simulink model "twoturbine"  (R2015b)
settings: Solver=VariableStepAuto  StartTime=0.0  StopTime=25  RelTol=1e-3
undefined symbols (not defined in the file): Ts
libraries: powerlib_meascontrol x4, powerlib x3, GE_275_103 x2
settings Model: SimulationMode=accelerator  Creator=Eren  LastModifiedBy=Eren

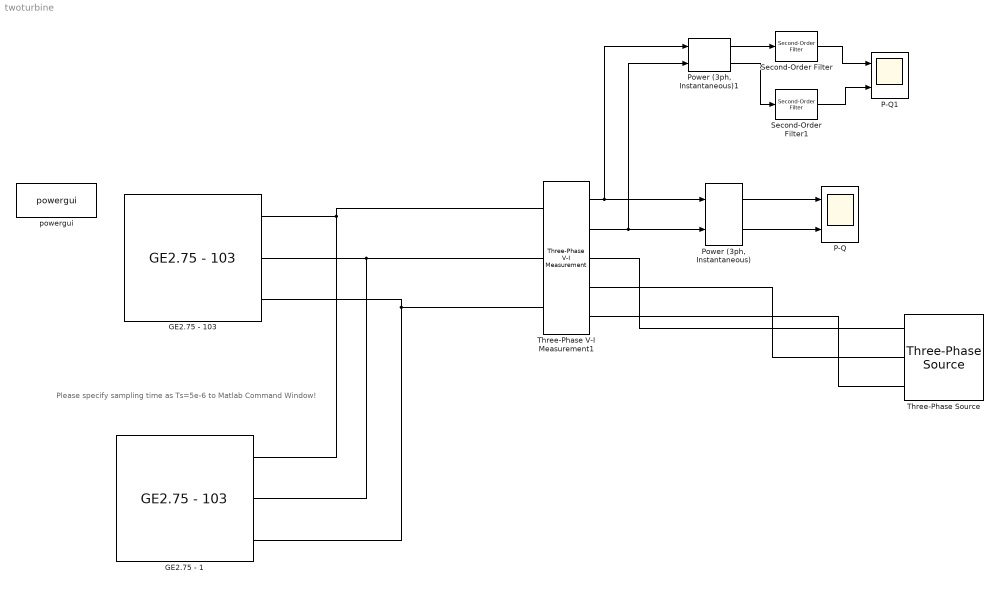
== system twoturbine ==
  note: Please specify sampling time as Ts=5e-6 to Matlab Command Window!
  GE2.75 - 1 : GE_275_103/GE2.75 - 103  Prated=2.75e6  R=51.5  windspeed=9  Jtotal=1058.2  p=1.225  startuptime=5  winit=-160  gear=117.4  wmax=2*pi*(1735/60)  fluxlinkage=4  pgen=2  Ld=10e-4  Lq=10.5e-4  Rs=1e-10  drivefreq=10e3  fnom=50  Srated=3.04e6  Vdcset=2500  Cdc=27e-3  Lfilter=2e-4
  GE2.75 - 103 : GE_275_103/GE2.75 - 103  Prated=2.75e6  R=51.5  windspeed=9  Jtotal=1058.2  p=1.225  startuptime=5  winit=-160  gear=117.4  wmax=2*pi*(1735/60)  fluxlinkage=4  pgen=2  Ld=10e-4  Lq=10.5e-4  Rs=1e-10  drivefreq=10e3  fnom=50  Srated=3.04e6  Vdcset=2500  Cdc=27e-3  Lfilter=2e-4
  P-Q : Scope  NumInputPorts=2
  P-Q1 : Scope  NumInputPorts=2
  "Power (3ph, Instantaneous)" : powerlib_meascontrol/Measurements/Power (3ph, Instantaneous)
  "Power (3ph, Instantaneous)1" : powerlib_meascontrol/Measurements/Power (3ph, Instantaneous)
  Second-Order Filter : powerlib_meascontrol/Filters/Second-Order Filter  FilterType=Lowpass  Fo=20  Zeta=0.707  Ts=0  Initialize=off  Vac_Init="[0,  0,  60]"  Vdc_Init=0  PlotResponse=off  FreqRange=[0, 500, 1]
  Second-Order Filter1 : powerlib_meascontrol/Filters/Second-Order Filter  FilterType=Lowpass  Fo=20  Zeta=0.707  Ts=0  Initialize=off  Vac_Init="[0,  0,  60]"  Vdc_Init=0  PlotResponse=off  FreqRange=[0, 500, 1]
  Three-Phase V-I Measurement1 : powerlib/Measurements/Three-Phase V-I Measurement  VoltageMeasurement=phase-to-ground  SetLabelV=off  LabelV=Vabc  Vpu=off  VpuLL=off  CurrentMeasurement=yes  SetLabelI=off  LabelI=Iabc  Ipu=off  Pbase=2.75e6  Vbase=690  OutputType=Complex  PhasorSimulation=off  PSBequivalent=0
  Three-Phase Source : powerlib/Electrical Sources/Three-Phase Source  InternalConnection=Yg  VoltagePhases=off  Voltage=690  PhaseAngle=0  Voltage_phases=[25e3 25e3 25e3]/sqrt(3)  PhaseAngles_phases=[0 -120 +120]  Frequency=50  NonIdealSource=on  SpecifyImpedance=off  Resistance=0  Inductance=0  ShortCircuitLevel=100e6  BaseVoltage=690  XRratio=7  BusType=swing  Pref=10e3  Qref=0  Prefabc=[10e3, 10e3, 10e3]  Qrefabc=[0, 0, 0]  Qmin=-inf  Qmax=inf
  powergui : powerlib/powergui  Priority=2  SimulationMode=Discrete  SolverType=Tustin  SampleTime=Ts  frequency=60  SPID=off  DisableSnubberDevices=off  DisableRonSwitches=off  DisableVfSwitches=off  SwTol=0  DisplayEquations=off  Interpol=off  ExternalGateDelay=off  methode=off  Ts=0  FunctionMessages=off  echomessages=off  HookPort=off  EnableUseOfTLC=off  x0status=blocks  frequencyindice=0  Pbase=100e6  ErrMax=1e-4  Iterations=50  UnitsV=kV  UnitsW=MW  buscounter=0  RestoreLinks=warning  ResistiveCurrentMeasurement=off  Frange=[0:2:500]  Ylog=off  Xlog=on  ShowGrid=off  save=off  variable=ZData  structure=0  ZoomFFT=on  StartTime=0.0  cycles=1  DisplayStyle=1  fundamental=60  FreqAxis=off  MaxFrequency=1000  frequencyindicesteady=1  RmsSteady=1  display=off
  wires:
  "Power (3ph, Instantaneous)"/1 -> P-Q/1
  Three-Phase V-I Measurement1/1 -> "Power (3ph, Instantaneous)"/1, "Power (3ph, Instantaneous)1"/1
  "Power (3ph, Instantaneous)"/2 -> P-Q/2
  Three-Phase V-I Measurement1/2 -> "Power (3ph, Instantaneous)1"/2, "Power (3ph, Instantaneous)"/2
  "Power (3ph, Instantaneous)1"/1 -> Second-Order Filter/1
  Second-Order Filter/1 -> P-Q1/1
  "Power (3ph, Instantaneous)1"/2 -> Second-Order Filter1/1
  Second-Order Filter1/1 -> P-Q1/2
  connections:
  GE2.75 - 103/RConn3 -- Three-Phase V-I Measurement1/LConn3 -- GE2.75 - 1/RConn3
  GE2.75 - 103/RConn1 -- GE2.75 - 1/RConn1 -- Three-Phase V-I Measurement1/LConn1
  GE2.75 - 103/RConn2 -- Three-Phase V-I Measurement1/LConn2 -- GE2.75 - 1/RConn2
  Three-Phase Source/RConn1 -- Three-Phase V-I Measurement1/RConn1
  Three-Phase Source/RConn2 -- Three-Phase V-I Measurement1/RConn2
  Three-Phase Source/RConn3 -- Three-Phase V-I Measurement1/RConn3
